simulink model "sm_forklift"  (R2021b)
settings: Solver=ode15s  StartTime=0.0  StopTime=53  MaxStep=1e-2  RelTol=1e-3  AbsTol=1e-3  EnableMultiTasking=on
model workspace: external: MATLAB File sm_forklift_parameters.m (data not in the file)
values from neighbouring files (symbols this model uses):
  g = 9.8    [sm_forklift_parameters.m]
undefined symbols (not defined in the file or in its folder): backRest, box, bump, chassis, fork, infPlane, main_mast, pulley, smiData, tire, top_mast, wheel, X, Y, Z
libraries: sm_lib x1413, nesl_utility x83, fl_lib x23, sm_backhoe_lib x6, SignalEditorBlockLib x1
(part 8 of 24)

== system sm_forklift/Warehouse/Racks/Rack 1/Rack End  ==
  Rack_AngleBrace_21_RIGID : Subsystem
  Rack_AngleBrace_22_RIGID : Subsystem
  Rack_AngleBrace_23_RIGID : Subsystem
  Rack_AngleBrace_24_RIGID : Subsystem
  Rack_AngleBrace_25_RIGID : Subsystem
  Rack_Leg_10_RIGID : Subsystem
  Rack_Leg_9_RIGID : Subsystem
  Rack_ShelfEnd_29_RIGID : Subsystem
  Rack_ShelfEnd_30_RIGID : Subsystem
  Rack_ShelfEnd_31_RIGID : Subsystem
  Rack_ShelfEnd_32_RIGID : Subsystem
  Rack_ShelfEnd_33_RIGID : Subsystem
  Rack_ShelfEnd_34_RIGID : Subsystem
  Rack_ShelfEnd_35_RIGID : Subsystem
  Conn1 : PMIOPort  Side=Left
  connections:
  Rack_AngleBrace_22_RIGID/LConn1 -- Rack_Leg_9_RIGID/LConn1 -- Rack_ShelfEnd_30_RIGID/LConn1 -- Rack_Leg_10_RIGID/LConn1 -- Rack_AngleBrace_25_RIGID/LConn1 -- Rack_AngleBrace_24_RIGID/LConn1 -- Rack_AngleBrace_23_RIGID/LConn1 -- Rack_AngleBrace_21_RIGID/LConn1 -- Rack_ShelfEnd_29_RIGID/LConn1 -- Rack_ShelfEnd_31_RIGID/LConn1 -- Rack_ShelfEnd_32_RIGID/LConn1 -- Rack_ShelfEnd_33_RIGID/LConn1 -- Rack_ShelfEnd_34_RIGID/LConn1 -- Rack_ShelfEnd_35_RIGID/LConn1
  Conn1/RConn1 -- Rack_ShelfEnd_29_RIGID/LConn2

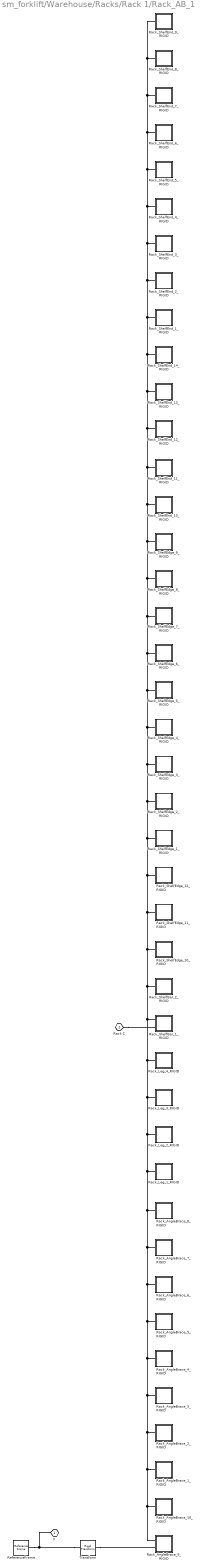
== system sm_forklift/Warehouse/Racks/Rack 1/Rack_AB_1 ==
  Rack_AngleBrace_10_RIGID : Subsystem
  Rack_AngleBrace_1_RIGID : Subsystem
  Rack_AngleBrace_2_RIGID : Subsystem
  Rack_AngleBrace_3_RIGID : Subsystem
  Rack_AngleBrace_4_RIGID : Subsystem
  Rack_AngleBrace_5_RIGID : Subsystem
  Rack_AngleBrace_6_RIGID : Subsystem
  Rack_AngleBrace_7_RIGID : Subsystem
  Rack_AngleBrace_8_RIGID : Subsystem
  Rack_AngleBrace_9_RIGID : Subsystem
  Rack_Leg_1_RIGID : Subsystem
  Rack_Leg_2_RIGID : Subsystem
  Rack_Leg_3_RIGID : Subsystem
  Rack_Leg_4_RIGID : Subsystem
  Rack_ShelfBar_1_RIGID : Subsystem
  Rack_ShelfBar_2_RIGID : Subsystem
  Rack_ShelfEdge_10_RIGID : Subsystem
  Rack_ShelfEdge_11_RIGID : Subsystem
  Rack_ShelfEdge_12_RIGID : Subsystem
  Rack_ShelfEdge_1_RIGID : Subsystem
  Rack_ShelfEdge_2_RIGID : Subsystem
  Rack_ShelfEdge_3_RIGID : Subsystem
  Rack_ShelfEdge_4_RIGID : Subsystem
  Rack_ShelfEdge_5_RIGID : Subsystem
  Rack_ShelfEdge_6_RIGID : Subsystem
  Rack_ShelfEdge_7_RIGID : Subsystem
  Rack_ShelfEdge_8_RIGID : Subsystem
  Rack_ShelfEdge_9_RIGID : Subsystem
  Rack_ShelfEnd_10_RIGID : Subsystem
  Rack_ShelfEnd_11_RIGID : Subsystem
  Rack_ShelfEnd_12_RIGID : Subsystem
  Rack_ShelfEnd_13_RIGID : Subsystem
  Rack_ShelfEnd_14_RIGID : Subsystem
  Rack_ShelfEnd_1_RIGID : Subsystem
  Rack_ShelfEnd_2_RIGID : Subsystem
  Rack_ShelfEnd_3_RIGID : Subsystem
  Rack_ShelfEnd_4_RIGID : Subsystem
  Rack_ShelfEnd_5_RIGID : Subsystem
  Rack_ShelfEnd_6_RIGID : Subsystem
  Rack_ShelfEnd_7_RIGID : Subsystem
  Rack_ShelfEnd_8_RIGID : Subsystem
  Rack_ShelfEnd_9_RIGID : Subsystem
  ReferenceFrame : sm_lib/Frames and Transforms/Reference Frame
  Transform : sm_lib/Frames and Transforms/Rigid Transform  TranslationMethod=Cartesian  TranslationStandardOffset=0  TranslationLengthUnit=m  TranslationStandardAxis=+Z  TranslationCartesianOffset=smiData.RigidTransform(197).translation  TranslationROffset=0  TranslationROffsetUnits=m  TranslationZOffset=0  TranslationZOffsetUnits=m  TranslationThetaOffset=0  TranslationThetaOffsetUnits=deg  RotationMethod=ArbitraryAxis  RotationAngleUnits=rad  RotationStandardAxis=+Z  RotationAngle=smiData.RigidTransform(197).angle  RotationArbitraryAxis=smiData.RigidTransform(197).axis  FollAlignAxisA=+X  BaseAlignAxisA=+Y  FollAlignAxisB=+Y  BaseAlignAxisB=+Z  RotationSequenceAxes=FollowerAxes  RotationSequence=XYX  RotationSequenceAngles=[0 0 0]  RotationSequenceAnglesUnits=deg  RotationMatrix=[1 0 0; 0 1 0; 0 0 1]
  F : PMIOPort  Side=Left
  Rack C : PMIOPort  Port=2  Side=Left
  connections:
  Rack_AngleBrace_1_RIGID/LConn1 -- Rack_ShelfEnd_8_RIGID/LConn1 -- Rack_ShelfEnd_9_RIGID/LConn1 -- Rack_ShelfEnd_7_RIGID/LConn1 -- Rack_ShelfEnd_6_RIGID/LConn1 -- Rack_ShelfEnd_5_RIGID/LConn1 -- Rack_ShelfEnd_4_RIGID/LConn1 -- Rack_ShelfEnd_3_RIGID/LConn1 -- Rack_ShelfEnd_2_RIGID/LConn1 -- Rack_ShelfEnd_1_RIGID/LConn1 -- Rack_ShelfEnd_14_RIGID/LConn1 -- Rack_ShelfEnd_13_RIGID/LConn1 -- Rack_ShelfEnd_12_RIGID/LConn1 -- Rack_ShelfEnd_11_RIGID/LConn1 -- Rack_ShelfEnd_10_RIGID/LConn1 -- Rack_ShelfEdge_9_RIGID/LConn1 -- Rack_ShelfEdge_8_RIGID/LConn1 -- Rack_ShelfEdge_7_RIGID/LConn1 -- Rack_ShelfEdge_6_RIGID/LConn1 -- Rack_ShelfEdge_5_RIGID/LConn1 -- Rack_ShelfEdge_4_RIGID/LConn1 -- Rack_ShelfEdge_3_RIGID/LConn1 -- Rack_ShelfEdge_2_RIGID/LConn1 -- Rack_ShelfEdge_1_RIGID/LConn1 -- Rack_ShelfEdge_12_RIGID/LConn1 -- Rack_ShelfEdge_11_RIGID/LConn1 -- Rack_ShelfEdge_10_RIGID/LConn1 -- Rack_ShelfBar_2_RIGID/LConn1 -- Rack_ShelfBar_1_RIGID/LConn1 -- Rack_Leg_4_RIGID/LConn1 -- Rack_Leg_3_RIGID/LConn1 -- Rack_Leg_2_RIGID/LConn1 -- Rack_Leg_1_RIGID/LConn1 -- Rack_AngleBrace_8_RIGID/LConn1 -- Rack_AngleBrace_7_RIGID/LConn1 -- Rack_AngleBrace_6_RIGID/LConn1 -- Rack_AngleBrace_5_RIGID/LConn1 -- Rack_AngleBrace_4_RIGID/LConn1 -- Rack_AngleBrace_3_RIGID/LConn1 -- Rack_AngleBrace_2_RIGID/LConn1 -- Rack_AngleBrace_10_RIGID/LConn1 -- Rack_AngleBrace_9_RIGID/LConn1
  Transform/RConn1 -- Rack_AngleBrace_9_RIGID/LConn2
  Transform/LConn1 -- F/RConn1 -- ReferenceFrame/RConn1
  Rack C/RConn1 -- Rack_ShelfBar_1_RIGID/LConn2

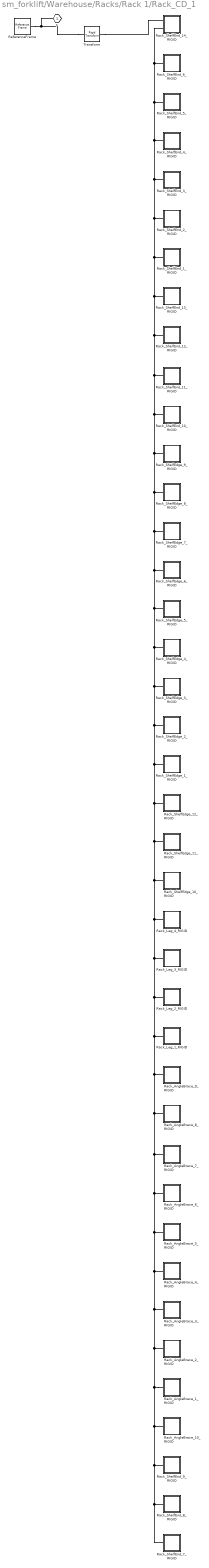
== system sm_forklift/Warehouse/Racks/Rack 1/Rack_CD_1 ==
  Rack_AngleBrace_10_RIGID : Subsystem
  Rack_AngleBrace_1_RIGID : Subsystem
  Rack_AngleBrace_2_RIGID : Subsystem
  Rack_AngleBrace_3_RIGID : Subsystem
  Rack_AngleBrace_4_RIGID : Subsystem
  Rack_AngleBrace_5_RIGID : Subsystem
  Rack_AngleBrace_6_RIGID : Subsystem
  Rack_AngleBrace_7_RIGID : Subsystem
  Rack_AngleBrace_8_RIGID : Subsystem
  Rack_AngleBrace_9_RIGID : Subsystem
  Rack_Leg_1_RIGID : Subsystem
  Rack_Leg_2_RIGID : Subsystem
  Rack_Leg_3_RIGID : Subsystem
  Rack_Leg_4_RIGID : Subsystem
  Rack_ShelfEdge_10_RIGID : Subsystem
  Rack_ShelfEdge_11_RIGID : Subsystem
  Rack_ShelfEdge_12_RIGID : Subsystem
  Rack_ShelfEdge_1_RIGID : Subsystem
  Rack_ShelfEdge_2_RIGID : Subsystem
  Rack_ShelfEdge_3_RIGID : Subsystem
  Rack_ShelfEdge_4_RIGID : Subsystem
  Rack_ShelfEdge_5_RIGID : Subsystem
  Rack_ShelfEdge_6_RIGID : Subsystem
  Rack_ShelfEdge_7_RIGID : Subsystem
  Rack_ShelfEdge_8_RIGID : Subsystem
  Rack_ShelfEdge_9_RIGID : Subsystem
  Rack_ShelfEnd_10_RIGID : Subsystem
  Rack_ShelfEnd_11_RIGID : Subsystem
  Rack_ShelfEnd_12_RIGID : Subsystem
  Rack_ShelfEnd_13_RIGID : Subsystem
  Rack_ShelfEnd_14_RIGID : Subsystem
  Rack_ShelfEnd_1_RIGID : Subsystem
  Rack_ShelfEnd_2_RIGID : Subsystem
  Rack_ShelfEnd_3_RIGID : Subsystem
  Rack_ShelfEnd_4_RIGID : Subsystem
  Rack_ShelfEnd_5_RIGID : Subsystem
  Rack_ShelfEnd_6_RIGID : Subsystem
  Rack_ShelfEnd_7_RIGID : Subsystem
  Rack_ShelfEnd_8_RIGID : Subsystem
  Rack_ShelfEnd_9_RIGID : Subsystem
  ReferenceFrame : sm_lib/Frames and Transforms/Reference Frame
  Transform : sm_lib/Frames and Transforms/Rigid Transform  TranslationMethod=Cartesian  TranslationStandardOffset=0  TranslationLengthUnit=m  TranslationStandardAxis=+Z  TranslationCartesianOffset=smiData.RigidTransform(193).translation  TranslationROffset=0  TranslationROffsetUnits=m  TranslationZOffset=0  TranslationZOffsetUnits=m  TranslationThetaOffset=0  TranslationThetaOffsetUnits=deg  RotationMethod=ArbitraryAxis  RotationAngleUnits=rad  RotationStandardAxis=+Z  RotationAngle=smiData.RigidTransform(193).angle  RotationArbitraryAxis=smiData.RigidTransform(193).axis  FollAlignAxisA=+X  BaseAlignAxisA=+Y  FollAlignAxisB=+Y  BaseAlignAxisB=+Z  RotationSequenceAxes=FollowerAxes  RotationSequence=XYX  RotationSequenceAngles=[0 0 0]  RotationSequenceAnglesUnits=deg  RotationMatrix=[1 0 0; 0 1 0; 0 0 1]
  F : PMIOPort  Side=Left
  connections:
  Rack_AngleBrace_1_RIGID/LConn1 -- Rack_ShelfEnd_14_RIGID/LConn2 -- Rack_ShelfEnd_6_RIGID/LConn1 -- Rack_ShelfEnd_5_RIGID/LConn1 -- Rack_ShelfEnd_4_RIGID/LConn1 -- Rack_ShelfEnd_3_RIGID/LConn1 -- Rack_ShelfEnd_2_RIGID/LConn1 -- Rack_ShelfEnd_1_RIGID/LConn1 -- Rack_ShelfEnd_13_RIGID/LConn1 -- Rack_ShelfEnd_12_RIGID/LConn1 -- Rack_ShelfEnd_11_RIGID/LConn1 -- Rack_ShelfEnd_10_RIGID/LConn1 -- Rack_ShelfEdge_9_RIGID/LConn1 -- Rack_ShelfEdge_8_RIGID/LConn1 -- Rack_ShelfEdge_7_RIGID/LConn1 -- Rack_ShelfEdge_6_RIGID/LConn1 -- Rack_ShelfEdge_5_RIGID/LConn1 -- Rack_ShelfEdge_4_RIGID/LConn1 -- Rack_ShelfEdge_3_RIGID/LConn1 -- Rack_ShelfEdge_2_RIGID/LConn1 -- Rack_ShelfEdge_1_RIGID/LConn1 -- Rack_ShelfEdge_12_RIGID/LConn1 -- Rack_ShelfEdge_11_RIGID/LConn1 -- Rack_ShelfEdge_10_RIGID/LConn1 -- Rack_Leg_4_RIGID/LConn1 -- Rack_Leg_3_RIGID/LConn1 -- Rack_Leg_2_RIGID/LConn1 -- Rack_Leg_1_RIGID/LConn1 -- Rack_AngleBrace_9_RIGID/LConn1 -- Rack_AngleBrace_8_RIGID/LConn1 -- Rack_AngleBrace_7_RIGID/LConn1 -- Rack_AngleBrace_6_RIGID/LConn1 -- Rack_AngleBrace_5_RIGID/LConn1 -- Rack_AngleBrace_4_RIGID/LConn1 -- Rack_AngleBrace_3_RIGID/LConn1 -- Rack_AngleBrace_2_RIGID/LConn1 -- Rack_AngleBrace_10_RIGID/LConn1 -- Rack_ShelfEnd_7_RIGID/LConn1 -- Rack_ShelfEnd_8_RIGID/LConn1 -- Rack_ShelfEnd_9_RIGID/LConn1
  Transform/RConn1 -- Rack_ShelfEnd_14_RIGID/LConn1
  Transform/LConn1 -- ReferenceFrame/RConn1 -- F/RConn1

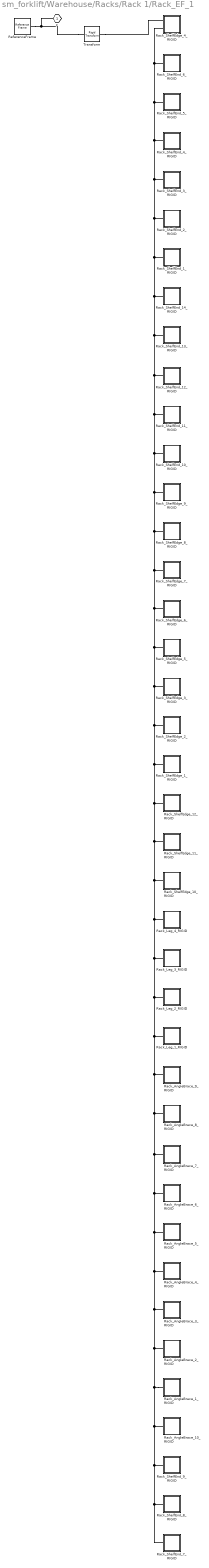
== system sm_forklift/Warehouse/Racks/Rack 1/Rack_EF_1 ==
  Rack_AngleBrace_10_RIGID : Subsystem
  Rack_AngleBrace_1_RIGID : Subsystem
  Rack_AngleBrace_2_RIGID : Subsystem
  Rack_AngleBrace_3_RIGID : Subsystem
  Rack_AngleBrace_4_RIGID : Subsystem
  Rack_AngleBrace_5_RIGID : Subsystem
  Rack_AngleBrace_6_RIGID : Subsystem
  Rack_AngleBrace_7_RIGID : Subsystem
  Rack_AngleBrace_8_RIGID : Subsystem
  Rack_AngleBrace_9_RIGID : Subsystem
  Rack_Leg_1_RIGID : Subsystem
  Rack_Leg_2_RIGID : Subsystem
  Rack_Leg_3_RIGID : Subsystem
  Rack_Leg_4_RIGID : Subsystem
  Rack_ShelfEdge_10_RIGID : Subsystem
  Rack_ShelfEdge_11_RIGID : Subsystem
  Rack_ShelfEdge_12_RIGID : Subsystem
  Rack_ShelfEdge_1_RIGID : Subsystem
  Rack_ShelfEdge_2_RIGID : Subsystem
  Rack_ShelfEdge_3_RIGID : Subsystem
  Rack_ShelfEdge_4_RIGID : Subsystem
  Rack_ShelfEdge_5_RIGID : Subsystem
  Rack_ShelfEdge_6_RIGID : Subsystem
  Rack_ShelfEdge_7_RIGID : Subsystem
  Rack_ShelfEdge_8_RIGID : Subsystem
  Rack_ShelfEdge_9_RIGID : Subsystem
  Rack_ShelfEnd_10_RIGID : Subsystem
  Rack_ShelfEnd_11_RIGID : Subsystem
  Rack_ShelfEnd_12_RIGID : Subsystem
  Rack_ShelfEnd_13_RIGID : Subsystem
  Rack_ShelfEnd_14_RIGID : Subsystem
  Rack_ShelfEnd_1_RIGID : Subsystem
  Rack_ShelfEnd_2_RIGID : Subsystem
  Rack_ShelfEnd_3_RIGID : Subsystem
  Rack_ShelfEnd_4_RIGID : Subsystem
  Rack_ShelfEnd_5_RIGID : Subsystem
  Rack_ShelfEnd_6_RIGID : Subsystem
  Rack_ShelfEnd_7_RIGID : Subsystem
  Rack_ShelfEnd_8_RIGID : Subsystem
  Rack_ShelfEnd_9_RIGID : Subsystem
  ReferenceFrame : sm_lib/Frames and Transforms/Reference Frame
  Transform : sm_lib/Frames and Transforms/Rigid Transform  TranslationMethod=Cartesian  TranslationStandardOffset=0  TranslationLengthUnit=m  TranslationStandardAxis=+Z  TranslationCartesianOffset=smiData.RigidTransform(195).translation  TranslationROffset=0  TranslationROffsetUnits=m  TranslationZOffset=0  TranslationZOffsetUnits=m  TranslationThetaOffset=0  TranslationThetaOffsetUnits=deg  RotationMethod=ArbitraryAxis  RotationAngleUnits=rad  RotationStandardAxis=+Z  RotationAngle=smiData.RigidTransform(195).angle  RotationArbitraryAxis=smiData.RigidTransform(195).axis  FollAlignAxisA=+X  BaseAlignAxisA=+Y  FollAlignAxisB=+Y  BaseAlignAxisB=+Z  RotationSequenceAxes=FollowerAxes  RotationSequence=XYX  RotationSequenceAngles=[0 0 0]  RotationSequenceAnglesUnits=deg  RotationMatrix=[1 0 0; 0 1 0; 0 0 1]
  F : PMIOPort  Side=Left
  connections:
  Rack_AngleBrace_1_RIGID/LConn1 -- Rack_ShelfEdge_4_RIGID/LConn2 -- Rack_ShelfEnd_6_RIGID/LConn1 -- Rack_ShelfEnd_5_RIGID/LConn1 -- Rack_ShelfEnd_4_RIGID/LConn1 -- Rack_ShelfEnd_3_RIGID/LConn1 -- Rack_ShelfEnd_2_RIGID/LConn1 -- Rack_ShelfEnd_1_RIGID/LConn1 -- Rack_ShelfEnd_14_RIGID/LConn1 -- Rack_ShelfEnd_13_RIGID/LConn1 -- Rack_ShelfEnd_12_RIGID/LConn1 -- Rack_ShelfEnd_11_RIGID/LConn1 -- Rack_ShelfEnd_10_RIGID/LConn1 -- Rack_ShelfEdge_9_RIGID/LConn1 -- Rack_ShelfEdge_8_RIGID/LConn1 -- Rack_ShelfEdge_7_RIGID/LConn1 -- Rack_ShelfEdge_6_RIGID/LConn1 -- Rack_ShelfEdge_5_RIGID/LConn1 -- Rack_ShelfEdge_3_RIGID/LConn1 -- Rack_ShelfEdge_2_RIGID/LConn1 -- Rack_ShelfEdge_1_RIGID/LConn1 -- Rack_ShelfEdge_12_RIGID/LConn1 -- Rack_ShelfEdge_11_RIGID/LConn1 -- Rack_ShelfEdge_10_RIGID/LConn1 -- Rack_Leg_4_RIGID/LConn1 -- Rack_Leg_3_RIGID/LConn1 -- Rack_Leg_2_RIGID/LConn1 -- Rack_Leg_1_RIGID/LConn1 -- Rack_AngleBrace_9_RIGID/LConn1 -- Rack_AngleBrace_8_RIGID/LConn1 -- Rack_AngleBrace_7_RIGID/LConn1 -- Rack_AngleBrace_6_RIGID/LConn1 -- Rack_AngleBrace_5_RIGID/LConn1 -- Rack_AngleBrace_4_RIGID/LConn1 -- Rack_AngleBrace_3_RIGID/LConn1 -- Rack_AngleBrace_2_RIGID/LConn1 -- Rack_AngleBrace_10_RIGID/LConn1 -- Rack_ShelfEnd_7_RIGID/LConn1 -- Rack_ShelfEnd_8_RIGID/LConn1 -- Rack_ShelfEnd_9_RIGID/LConn1
  Transform/RConn1 -- Rack_ShelfEdge_4_RIGID/LConn1
  Transform/LConn1 -- ReferenceFrame/RConn1 -- F/RConn1
